simulink model "Final_Project_EEM_EKF_SIM"  (R2020a)
settings: Solver=ode45  StartTime=0  StopTime=t_runtime  FixedStep=clockt/4  RelTol=1e-3  AbsTol=1e-6
PreLoadFcn:
  | run(fullfile('Final_Project_EEM_SIM_init_params.m'));
StopFcn:
  | run('EKF_Simulation_Run_Plots_EEM.m');
values from neighbouring files (symbols this model uses):
  alph1 = Force*L_arm/I1    (= 0.055)    [Final_Project_EEM_SIM_init_params.m]
  alphs1 = 0.1*alph1    (= 0.0055)    [Final_Project_EEM_SIM_init_params.m]
  alphsu = 0.1*alphu    [Final_Project_EEM_SIM_init_params.m]
  alphsv = 0.1*alphv    [Final_Project_EEM_SIM_init_params.m]
  alphu = [sqrt(2) sqrt(2)]/2*[alph2 alph3]'    [Final_Project_EEM_SIM_init_params.m]
  alphv = [-sqrt(2) sqrt(2)]/2*[alph2 alph3]'    [Final_Project_EEM_SIM_init_params.m]
  clockt = 1/200    (= 0.005)    [Final_Project_EEM_SIM_init_params.m]
  DB = 0.345*pi/180    (= 0.00602138591938)    [Final_Project_EEM_SIM_init_params.m]
  delt = .1    (= 0.1)    [Final_Project_EEM_SIM_init_params.m]
  euler_0 = [-30 -10 -60]    [Final_Project_EEM_SIM_init_params.m]
  f_moon = .0012    (= 0.0012)    [Final_Project_EEM_SIM_init_params.m]
  Force = 100    [Final_Project_EEM_SIM_init_params.m]
  Inertia_0 = diag([I2,I3,I1],0)    [Final_Project_EEM_SIM_init_params.m]
  L_arm = 5.5    [Final_Project_EEM_SIM_init_params.m]
  lla_0 = [0.6, 23, 50000]    [Final_Project_EEM_SIM_init_params.m]
  mass_0 = 33296    [Final_Project_EEM_SIM_init_params.m]
  omega_moon = 2.7e-6    (= 2.7e-06)    [Final_Project_EEM_SIM_init_params.m]
  pqr_0 = [0.5730    0.5730    6.8080]    [Final_Project_EEM_SIM_init_params.m]
  r_moon_eq = 5702428    [Final_Project_EEM_SIM_init_params.m]
  tmin = 0.014    [Final_Project_EEM_SIM_init_params.m]
  vel_0 = angle2dcm(euler_0(3)*pi/180, euler_0(2)*pi/180, euler_0(1)*pi/180, 'ZYX')*vel    [Final_Project_EEM_SIM_init_params.m]
undefined symbols (not defined in the file or in its folder): deg, e0_0, e1_0, e2_0, e3_0, Newton, rad, Raphson, s
libraries: sharedtransform x5, sharedutil x5, aerolibtransform2 x4, shared6dofsys x3, aerolibconvert2 x3, vrlib x2, aerolibutil x1, aerolibgravity2 x1, aero_libdap x1
(part 2 of 3)

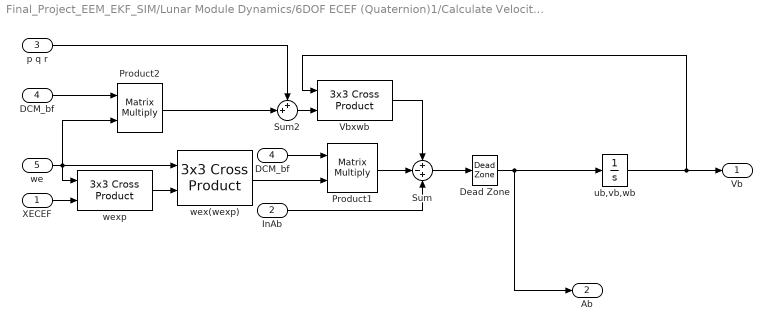
== system Final_Project_EEM_EKF_SIM/Lunar Module Dynamics/6DOF ECEF (Quaternion)1/Calculate Velocity in Body Axes ==
  XECEF : Inport
  InAb : Inport  Port=2
  p q r : Inport  Port=3
  DCM_bf : Inport  Port=4
  we : Inport  Port=5
  "DCM_bf " : InportShadow  Port=4
  Dead Zone : DeadZone  LowerValue=-eps  UpperValue=eps  SaturateOnIntegerOverflow=on
  Product1 : Product  Multiplication=Matrix(*)  RndMeth=Zero
  Product2 : Product  Multiplication=Matrix(*)  RndMeth=Zero
  Sum : Sum  Inputs=+-+  SaturateOnIntegerOverflow=on
  Sum2 : Sum  Inputs=++|  SaturateOnIntegerOverflow=on
  Vbxwb : sharedutil/3x3 Cross Product  aMode=aMode
      settings: SourceProductBaseCode=AE,PW,MT,VE,VP
  ub,vb,wb : Integrator  InitialCondition=Vm_0  ContinuousStateAttributes=Vm_statename
  wex(wexp) : sharedutil/3x3 Cross Product  aMode=aMode
      settings: SourceProductBaseCode=AE,PW,MT,VE,VP
  wexp : sharedutil/3x3 Cross Product  aMode=aMode
      settings: SourceProductBaseCode=AE,PW,MT,VE,VP
  Vb : Outport  VectorParamsAs1DForOutWhenUnconnected=off
  Ab : Outport  Port=2  PortDimensions=3  VectorParamsAs1DForOutWhenUnconnected=off
  wires:
  DCM_bf/1 -> Product1/1
  we/1 -> wex(wexp)/1, wexp/1, Product2/2
  InAb/1 -> Sum/3
  Vbxwb/1 -> Sum/1
  XECEF/1 -> wexp/2
  wex(wexp)/1 -> Product1/2
  wexp/1 -> wex(wexp)/2
  Product2/1 -> Sum2/2
  Sum2/1 -> Vbxwb/2
  Product1/1 -> Sum/2
  Sum/1 -> Dead Zone/1
  ub,vb,wb/1 -> Vbxwb/1, Vb/1
  "DCM_bf "/1 -> Product2/1
  p q r/1 -> Sum2/1
  Dead Zone/1 -> ub,vb,wb/1, Ab/1

== system Final_Project_EEM_EKF_SIM/Lunar Module Dynamics/6DOF ECEF (Quaternion)1/Celestial Longitude of Greenwich ==
  Initial Angle : Inport  Unit=rad
  Constant1 : Constant  Value=w_E
  Integrator : Integrator  ContinuousStateAttributes=LG_statename
  Sum : Sum  Inputs=|++
  Lambda : Outport  VectorParamsAs1DForOutWhenUnconnected=off
  wires:
  Initial Angle/1 -> Sum/1
  Integrator/1 -> Sum/2
  Constant1/1 -> Integrator/1  "we"
  Sum/1 -> Lambda/1

== system Final_Project_EEM_EKF_SIM/Lunar Module Dynamics/6DOF ECEF (Quaternion)1/ECEF to Inertial ==
  LG : Inport
  Create 3x3 Matrix : sharedutil/Create 3x3 Matrix  aMode=aMode
      settings: SourceProductBaseCode=AE,PW,MT,VE,VP
  Unary Minus : UnaryMinus
  Zero : Constant  Value=0
  Zero1 : Constant
  sincos : Trigonometry  Operator=sincos
  DCM_IF : Outport  VectorParamsAs1DForOutWhenUnconnected=off
  wires:
  LG/1 -> sincos/1
  Create 3x3 Matrix/1 -> DCM_IF/1
  Zero1/1 -> Create 3x3 Matrix/9
  Zero/1 -> Create 3x3 Matrix/8, Create 3x3 Matrix/7, Create 3x3 Matrix/6, Create 3x3 Matrix/3
  sincos/2 -> Create 3x3 Matrix/1, Create 3x3 Matrix/5
  sincos/1 -> Create 3x3 Matrix/4, Unary Minus/1
  Unary Minus/1 -> Create 3x3 Matrix/2

== system Final_Project_EEM_EKF_SIM/Lunar Module Dynamics/6DOF ECEF (Quaternion)1/Velocity Conversion ==
  in : Inport  Unit=ft/s
  Unit Conversion : UnitConversion
  out : Outport  VectorParamsAs1DForOutWhenUnconnected=off
  wires:
  in/1 -> Unit Conversion/1
  Unit Conversion/1 -> out/1

== system Final_Project_EEM_EKF_SIM/Lunar Module Dynamics/6DOF ECEF (Quaternion)1/Velocity Conversion1 ==
  in : Inport  Unit=ft/sec^2
  Unit Conversion : UnitConversion
  out : Outport  VectorParamsAs1DForOutWhenUnconnected=off
  wires:
  in/1 -> Unit Conversion/1
  Unit Conversion/1 -> out/1

== system Final_Project_EEM_EKF_SIM/Lunar Module Dynamics/6DOF ECEF (Quaternion)1/Velocity Conversion2 ==
  in : Inport  Unit=ft/s
  Unit Conversion : UnitConversion
  out : Outport  Unit=ft/s  VectorParamsAs1DForOutWhenUnconnected=off
  wires:
  in/1 -> Unit Conversion/1
  Unit Conversion/1 -> out/1

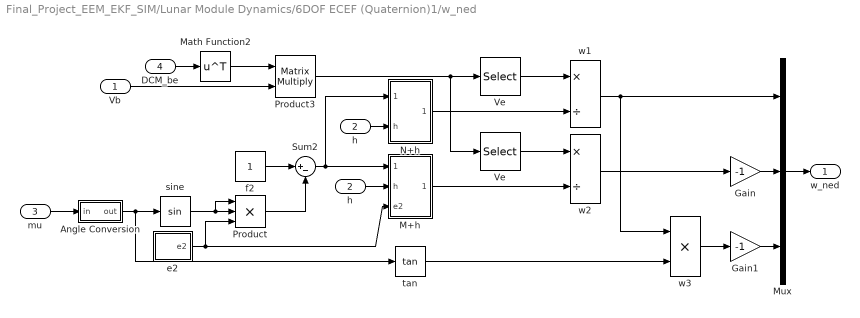
== system Final_Project_EEM_EKF_SIM/Lunar Module Dynamics/6DOF ECEF (Quaternion)1/w_ned ==
  Vb : Inport
  h : Inport  Port=2
  mu : Inport  Port=3
  DCM_be : Inport  Port=4
  Angle Conversion : Subsystem
  Gain : Gain  Gain=-1
  Gain1 : Gain  Gain=-1
  M+h : Subsystem
  Math Function2 : Math  Operator=transpose  SignedPower=on  SaturateOnIntegerOverflow=on
  Mux : Mux  Inputs=3
  N+h : Subsystem
  Product : Product  Inputs=3  RndMeth=Zero
  Product3 : Product  Multiplication=Matrix(*)  RndMeth=Zero
  Sum2 : Sum  Inputs=|+-
  Ve : Selector  InputPortWidth=3  IndexOptions=Index vector (dialog)  Indices=2  OutputSizes=1
  "Ve " : Selector  InputPortWidth=3  IndexOptions=Index vector (dialog)  Indices=1  OutputSizes=1
  e2 : Subsystem
  f2 : Constant
  "h " : InportShadow  Port=2
  sine : Trigonometry
  tan : Trigonometry  Operator=tan
  w1 : Product  Inputs=*/
  w2 : Product  Inputs=*/
  w3 : Product  Inputs=**
  w_ned : Outport  VectorParamsAs1DForOutWhenUnconnected=off
  wires:
  Angle Conversion/1(out) -> sine/1, tan/1
  Math Function2/1 -> Product3/1
  Vb/1 -> Product3/2
  DCM_be/1 -> Math Function2/1
  "h "/1 -> N+h/2(h)
  h/1 -> M+h/2(h)
  Product3/1 -> Ve/1, "Ve "/1
  mu/1 -> Angle Conversion/1(in)
  e2/1(e2) -> Product/3, M+h/3(e2)
  sine/1 -> Product/2, Product/1
  Product/1 -> Sum2/2
  f2/1 -> Sum2/1
  Sum2/1 -> N+h/1(den), M+h/1(den)
  Ve/1 -> w1/1
  N+h/1(N+h) -> w1/2
  "Ve "/1 -> w2/1
  M+h/1(M+h) -> w2/2
  w2/1 -> Gain/1
  tan/1 -> w3/2
  w1/1 -> w3/1, Mux/1
  w3/1 -> Gain1/1
  Gain/1 -> Mux/2
  Gain1/1 -> Mux/3
  Mux/1 -> w_ned/1

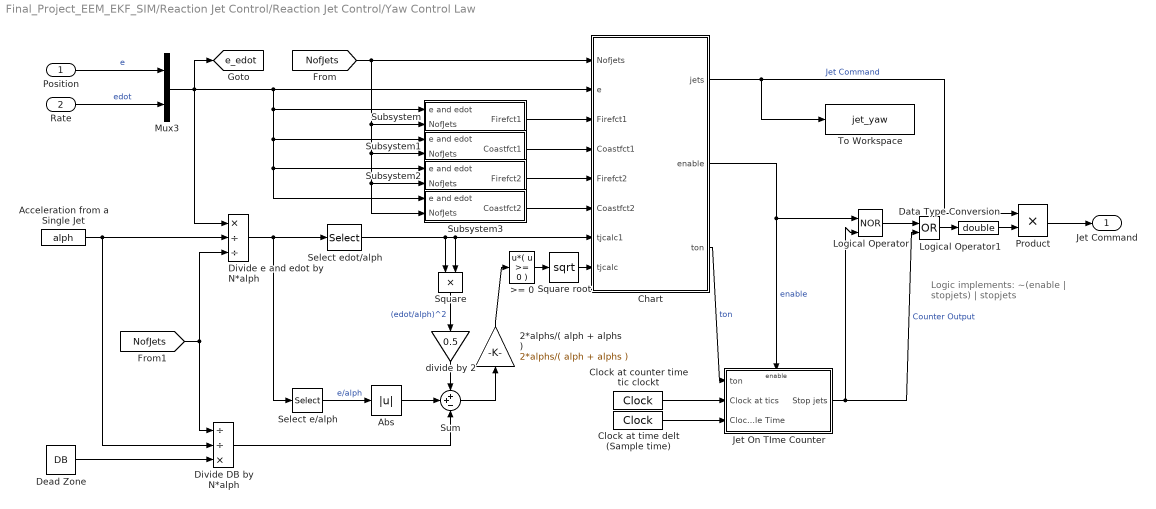
== system Final_Project_EEM_EKF_SIM/Reaction Jet Control/Reaction Jet Control/Yaw Control Law ==
  note: Logic implements:
      | ~(enable | stopjets) | stopjets
  Position : Inport  Unit=rad
  Rate : Inport  Port=2  Unit=rad/sec
  2*alphs/( alph + alphs ) : Gain  Gain=2*alphs/( alph + alphs )  SaturateOnIntegerOverflow=on  OutDataTypeStr=Inherit: Same as input  ParamDataTypeStr=Inherit: Same as input
  >= 0 : Fcn  Expr=u*( u >= 0 )
  Abs : Abs  SaturateOnIntegerOverflow=on
  Acceleration from a Single Jet : Constant  Value=alph
  Chart : Stateflow chart  TreatAsAtomicUnit=on
  Clock at counter time tic clockt : DigitalClock  SampleTime=clockt
  Clock at time delt (Sample time) : DigitalClock  SampleTime=delt
  Data Type Conversion : DataTypeConversion  OutDataTypeStr=double
  Dead Zone : Constant  Value=DB
  Divide e and edot by N*alph : Product  Inputs=*//  InputSameDT=on  RndMeth=Zero  SaturateOnIntegerOverflow=on  OutDataTypeStr=Inherit: Same as first input
  Divide DB by N*alph : Product  Inputs=//*  InputSameDT=on  RndMeth=Zero  SaturateOnIntegerOverflow=on  OutDataTypeStr=Inherit: Same as first input
  Jet On TIme Counter : Subsystem  TreatAsAtomicUnit=on
  Logical Operator : Logic  Operator=NOR  IconShape=distinctive  OutDataTypeStr=boolean
  Logical Operator1 : Logic  Operator=OR  IconShape=distinctive  OutDataTypeStr=boolean
  Mux3 : Mux  Inputs=2
  Product : Product  InputSameDT=on  RndMeth=Zero  SaturateOnIntegerOverflow=on  OutDataTypeStr=Inherit: Same as first input
  Select e/alph : Selector  InputPortWidth=2  IndexOptions=Index vector (dialog)  Indices=[1]  OutputSizes=1
  Select edot/alph : Selector  InputPortWidth=2  IndexOptions=Index vector (dialog)  Indices=[2]  OutputSizes=1
  Square : Product  InputSameDT=on  RndMeth=Zero  SaturateOnIntegerOverflow=on  OutDataTypeStr=Inherit: Same as first input
  Square root : Math  Operator=sqrt  SignedPower=on  SaturateOnIntegerOverflow=on
  Subsystem : Subsystem
  Subsystem1 : Subsystem
  Subsystem2 : Subsystem
  Subsystem3 : Subsystem
  Sum : Sum  Inputs=++-  InputSameDT=on  SaturateOnIntegerOverflow=on  OutDataTypeStr=Inherit: Same as first input
  To Workspace : ToWorkspace  VariableName=jet_yaw  SaveFormat=Timeseries  SampleTime=-1
  divide by 2 : Gain  Gain=0.5  SaturateOnIntegerOverflow=on  OutDataTypeStr=Inherit: Same as input  ParamDataTypeStr=Inherit: Same as input
  Jet Command : Outport  Unit=lbf  InitialOutput=0  VectorParamsAs1DForOutWhenUnconnected=off
  tag scope: e_edot=global
  wires:
  Data Type Conversion/1 -> Product/2
  >= 0/1 -> Square root/1
  2*alphs/( alph + alphs )/1 -> >= 0/1
  [NofJets] -> Subsystem3/2(NofJets), Subsystem2/2(NofJets), Subsystem1/2(NofJets), Subsystem/2(NofJets), Chart/1(Nofjets)
  Rate/1 -> Mux3/2  "edot"
  Position/1 -> Mux3/1  "e"
  Mux3/1 -> Divide e and edot by N*alph/1, Subsystem/1(e and edot), Subsystem1/1(e and edot), Subsystem2/1(e and edot), Subsystem3/1(e and edot), Chart/2(e), [e_edot]
  Square/1 -> divide by 2/1  "(edot/alph)^2"
  Square root/1 -> Chart/8(tjcalc)
  Chart/1(jets) -> To Workspace/1, Product/1  "Jet Command"
  Select edot/alph/1 -> Square/1, Chart/7(tjcalc1), Square/2
  Select e/alph/1 -> Abs/1  "e/alph"
  divide by 2/1 -> Sum/1
  Sum/1 -> 2*alphs/( alph + alphs )/1
  Abs/1 -> Sum/2
  Divide e and edot by N*alph/1 -> Select edot/alph/1, Select e/alph/1
  [NofJets] -> Divide e and edot by N*alph/3, Divide DB by N*alph/1
  Acceleration from a Single Jet/1 -> Divide DB by N*alph/2, Divide e and edot by N*alph/2
  Dead Zone/1 -> Divide DB by N*alph/3
  Divide DB by N*alph/1 -> Sum/3
  Chart/2(enable) -> Jet On TIme Counter/Enable, Logical Operator/1  "enable"
  Logical Operator1/1 -> Data Type Conversion/1
  Chart/3(ton) -> Jet On TIme Counter/1(ton)  "ton"
  Clock at counter time tic clockt/1 -> Jet On TIme Counter/2(Clock at tics)
  Clock at time delt (Sample time)/1 -> Jet On TIme Counter/3(Clock at Sample Time)
  Jet On TIme Counter/1(Stop jets) -> Logical Operator/2, Logical Operator1/2  "Counter Output"
  Logical Operator/1 -> Logical Operator1/1
  Subsystem3/1(Coastfct2) -> Chart/6(Coastfct2)
  Subsystem2/1(Firefct2) -> Chart/5(Firefct2)
  Subsystem1/1(Coastfct1) -> Chart/4(Coastfct1)
  Subsystem/1(Firefct1) -> Chart/3(Firefct1)
  Product/1 -> Jet Command/1

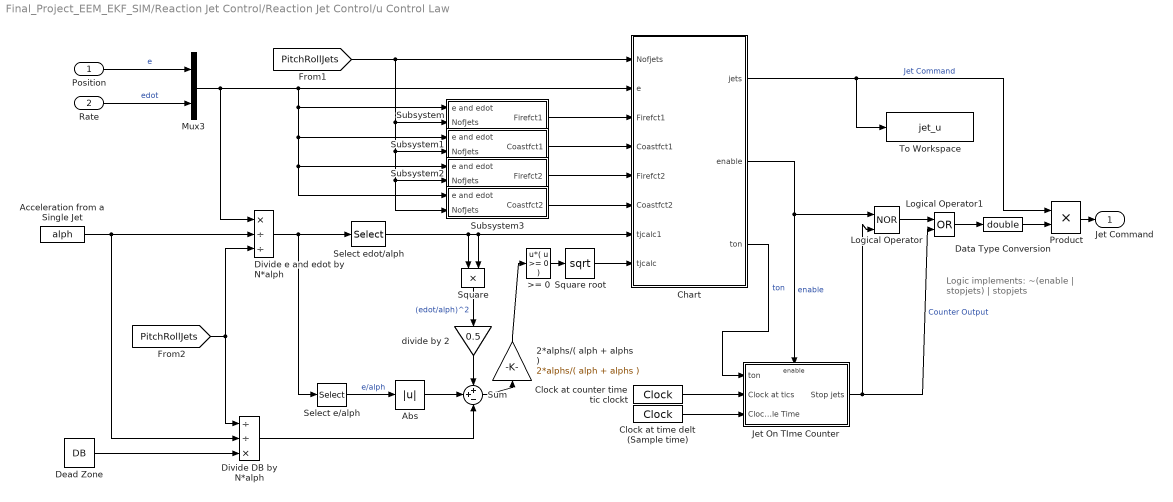
== system Final_Project_EEM_EKF_SIM/Reaction Jet Control/Reaction Jet Control/u Control Law ==
  note: Logic implements:
      | ~(enable | stopjets) | stopjets
  Position : Inport  Unit=rad
  Rate : Inport  Port=2  Unit=rad/sec
  2*alphs/( alph + alphs ) : Gain  Gain=2*alphs/( alph + alphs )  SaturateOnIntegerOverflow=on  OutDataTypeStr=Inherit: Same as input  ParamDataTypeStr=Inherit: Same as input
  >= 0 : Fcn  Expr=u*( u >= 0 )
  Abs : Abs  SaturateOnIntegerOverflow=on
  Acceleration from a Single Jet : Constant  Value=alph
  Chart : Stateflow chart  TreatAsAtomicUnit=on
  Clock at counter time tic clockt : DigitalClock  SampleTime=clockt
  Clock at time delt (Sample time) : DigitalClock  SampleTime=delt
  Data Type Conversion : DataTypeConversion  OutDataTypeStr=double
  Dead Zone : Constant  Value=DB
  Divide e and edot by N*alph : Product  Inputs=*//  InputSameDT=on  RndMeth=Zero  SaturateOnIntegerOverflow=on  OutDataTypeStr=Inherit: Same as first input
  Divide DB by N*alph : Product  Inputs=//*  InputSameDT=on  RndMeth=Zero  SaturateOnIntegerOverflow=on  OutDataTypeStr=Inherit: Same as first input
  Jet On TIme Counter : Subsystem  TreatAsAtomicUnit=on
  Logical Operator : Logic  Operator=NOR  IconShape=distinctive  OutDataTypeStr=boolean
  Logical Operator1 : Logic  Operator=OR  IconShape=distinctive  OutDataTypeStr=boolean
  Mux3 : Mux  Inputs=2
  Product : Product  InputSameDT=on  RndMeth=Zero  SaturateOnIntegerOverflow=on  OutDataTypeStr=Inherit: Same as first input
  Select e/alph : Selector  InputPortWidth=2  IndexOptions=Index vector (dialog)  Indices=[1]  OutputSizes=1
  Select edot/alph : Selector  InputPortWidth=2  IndexOptions=Index vector (dialog)  Indices=[2]  OutputSizes=1
  Square : Product  InputSameDT=on  RndMeth=Zero  SaturateOnIntegerOverflow=on  OutDataTypeStr=Inherit: Same as first input
  Square root : Math  Operator=sqrt  SignedPower=on  SaturateOnIntegerOverflow=on
  Subsystem : Subsystem
  Subsystem1 : Subsystem
  Subsystem2 : Subsystem
  Subsystem3 : Subsystem
  Sum : Sum  Inputs=++-  InputSameDT=on  SaturateOnIntegerOverflow=on  OutDataTypeStr=Inherit: Same as first input
  To Workspace : ToWorkspace  VariableName=jet_u  SaveFormat=Timeseries  SampleTime=-1
  divide by 2 : Gain  Gain=0.5  SaturateOnIntegerOverflow=on  OutDataTypeStr=Inherit: Same as input  ParamDataTypeStr=Inherit: Same as input
  Jet Command : Outport  Unit=lbf  InitialOutput=0  VectorParamsAs1DForOutWhenUnconnected=off
  wires:
  Data Type Conversion/1 -> Product/2
  >= 0/1 -> Square root/1
  2*alphs/( alph + alphs )/1 -> >= 0/1
  Product/1 -> Jet Command/1
  Subsystem/1(Firefct1) -> Chart/3(Firefct1)
  Subsystem1/1(Coastfct1) -> Chart/4(Coastfct1)
  Subsystem2/1(Firefct2) -> Chart/5(Firefct2)
  Subsystem3/1(Coastfct2) -> Chart/6(Coastfct2)
  Logical Operator/1 -> Logical Operator1/1
  Jet On TIme Counter/1(Stop jets) -> Logical Operator1/2, Logical Operator/2  "Counter Output"
  Clock at time delt (Sample time)/1 -> Jet On TIme Counter/3(Clock at Sample Time)
  Clock at counter time tic clockt/1 -> Jet On TIme Counter/2(Clock at tics)
  Chart/3(ton) -> Jet On TIme Counter/1(ton)  "ton"
  Logical Operator1/1 -> Data Type Conversion/1
  Chart/2(enable) -> Jet On TIme Counter/Enable, Logical Operator/1  "enable"
  Divide DB by N*alph/1 -> Sum/3
  Dead Zone/1 -> Divide DB by N*alph/3
  Acceleration from a Single Jet/1 -> Divide DB by N*alph/2, Divide e and edot by N*alph/2
  [PitchRollJets] -> Divide DB by N*alph/1, Divide e and edot by N*alph/3
  Divide e and edot by N*alph/1 -> Select e/alph/1, Select edot/alph/1
  Abs/1 -> Sum/2
  Sum/1 -> 2*alphs/( alph + alphs )/1
  divide by 2/1 -> Sum/1
  Select e/alph/1 -> Abs/1  "e/alph"
  Select edot/alph/1 -> Square/2, Chart/7(tjcalc1), Square/1
  Square root/1 -> Chart/8(tjcalc)
  Square/1 -> divide by 2/1  "(edot/alph)^2"
  Mux3/1 -> Divide e and edot by N*alph/1, Subsystem3/1(e and edot), Subsystem2/1(e and edot), Subsystem1/1(e and edot), Subsystem/1(e and edot), Chart/2(e)
  Position/1 -> Mux3/1  "e"
  Rate/1 -> Mux3/2  "edot"
  [PitchRollJets] -> Chart/1(Nofjets), Subsystem/2(NofJets), Subsystem1/2(NofJets), Subsystem2/2(NofJets), Subsystem3/2(NofJets)
  Chart/1(jets) -> To Workspace/1, Product/1  "Jet Command"

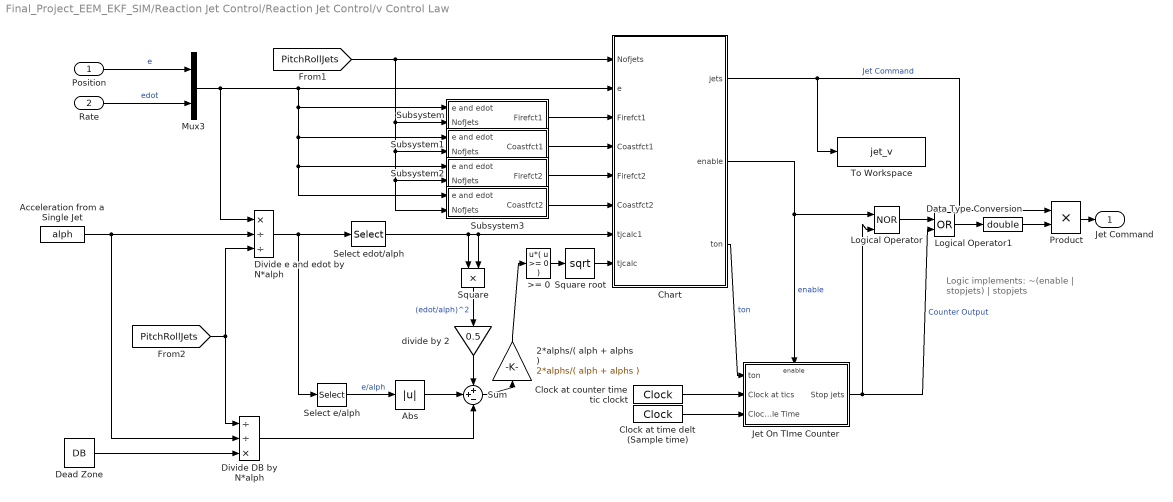
== system Final_Project_EEM_EKF_SIM/Reaction Jet Control/Reaction Jet Control/v Control Law ==
  note: Logic implements:
      | ~(enable | stopjets) | stopjets
  Position : Inport  Unit=rad
  Rate : Inport  Port=2  Unit=rad/sec
  2*alphs/( alph + alphs ) : Gain  Gain=2*alphs/( alph + alphs )  SaturateOnIntegerOverflow=on  OutDataTypeStr=Inherit: Same as input  ParamDataTypeStr=Inherit: Same as input
  >= 0 : Fcn  Expr=u*( u >= 0 )
  Abs : Abs  SaturateOnIntegerOverflow=on
  Acceleration from a Single Jet : Constant  Value=alph
  Chart : Stateflow chart  TreatAsAtomicUnit=on
  Clock at counter time tic clockt : DigitalClock  SampleTime=clockt
  Clock at time delt (Sample time) : DigitalClock  SampleTime=delt
  Data Type Conversion : DataTypeConversion  OutDataTypeStr=double
  Dead Zone : Constant  Value=DB
  Divide e and edot by N*alph : Product  Inputs=*//  InputSameDT=on  RndMeth=Zero  SaturateOnIntegerOverflow=on  OutDataTypeStr=Inherit: Same as first input
  Divide DB by N*alph : Product  Inputs=//*  InputSameDT=on  RndMeth=Zero  SaturateOnIntegerOverflow=on  OutDataTypeStr=Inherit: Same as first input
  Jet On TIme Counter : Subsystem  TreatAsAtomicUnit=on
  Logical Operator : Logic  Operator=NOR  IconShape=distinctive  OutDataTypeStr=boolean
  Logical Operator1 : Logic  Operator=OR  IconShape=distinctive  OutDataTypeStr=boolean
  Mux3 : Mux  Inputs=2
  Product : Product  InputSameDT=on  RndMeth=Zero  SaturateOnIntegerOverflow=on  OutDataTypeStr=Inherit: Same as first input
  Select e/alph : Selector  InputPortWidth=2  IndexOptions=Index vector (dialog)  Indices=[1]  OutputSizes=1
  Select edot/alph : Selector  InputPortWidth=2  IndexOptions=Index vector (dialog)  Indices=[2]  OutputSizes=1
  Square : Product  InputSameDT=on  RndMeth=Zero  SaturateOnIntegerOverflow=on  OutDataTypeStr=Inherit: Same as first input
  Square root : Math  Operator=sqrt  SignedPower=on  SaturateOnIntegerOverflow=on
  Subsystem : Subsystem
  Subsystem1 : Subsystem
  Subsystem2 : Subsystem
  Subsystem3 : Subsystem
  Sum : Sum  Inputs=++-  InputSameDT=on  SaturateOnIntegerOverflow=on  OutDataTypeStr=Inherit: Same as first input
  To Workspace : ToWorkspace  VariableName=jet_v  SaveFormat=Timeseries  SampleTime=-1
  divide by 2 : Gain  Gain=0.5  SaturateOnIntegerOverflow=on  OutDataTypeStr=Inherit: Same as input  ParamDataTypeStr=Inherit: Same as input
  Jet Command : Outport  Unit=lbf  InitialOutput=0  VectorParamsAs1DForOutWhenUnconnected=off
  wires:
  Data Type Conversion/1 -> Product/2
  >= 0/1 -> Square root/1
  2*alphs/( alph + alphs )/1 -> >= 0/1
  Product/1 -> Jet Command/1
  Subsystem/1(Firefct1) -> Chart/3(Firefct1)
  Subsystem1/1(Coastfct1) -> Chart/4(Coastfct1)
  Subsystem2/1(Firefct2) -> Chart/5(Firefct2)
  Subsystem3/1(Coastfct2) -> Chart/6(Coastfct2)
  Logical Operator/1 -> Logical Operator1/1
  Jet On TIme Counter/1(Stop jets) -> Logical Operator1/2, Logical Operator/2  "Counter Output"
  Clock at time delt (Sample time)/1 -> Jet On TIme Counter/3(Clock at Sample Time)
  Clock at counter time tic clockt/1 -> Jet On TIme Counter/2(Clock at tics)
  Chart/3(ton) -> Jet On TIme Counter/1(ton)  "ton"
  Logical Operator1/1 -> Data Type Conversion/1
  Chart/2(enable) -> Logical Operator/1, Jet On TIme Counter/Enable  "enable"
  Divide DB by N*alph/1 -> Sum/3
  Dead Zone/1 -> Divide DB by N*alph/3
  Acceleration from a Single Jet/1 -> Divide DB by N*alph/2, Divide e and edot by N*alph/2
  [PitchRollJets] -> Divide DB by N*alph/1, Divide e and edot by N*alph/3
  Divide e and edot by N*alph/1 -> Select e/alph/1, Select edot/alph/1
  Abs/1 -> Sum/2
  Sum/1 -> 2*alphs/( alph + alphs )/1
  divide by 2/1 -> Sum/1
  Select e/alph/1 -> Abs/1  "e/alph"
  Select edot/alph/1 -> Square/2, Chart/7(tjcalc1), Square/1
  Chart/1(jets) -> To Workspace/1, Product/1  "Jet Command"
  Square root/1 -> Chart/8(tjcalc)
  Square/1 -> divide by 2/1  "(edot/alph)^2"
  Mux3/1 -> Divide e and edot by N*alph/1, Subsystem3/1(e and edot), Subsystem2/1(e and edot), Subsystem1/1(e and edot), Subsystem/1(e and edot), Chart/2(e)
  Position/1 -> Mux3/1  "e"
  Rate/1 -> Mux3/2  "edot"
  [PitchRollJets] -> Chart/1(Nofjets), Subsystem/2(NofJets), Subsystem1/2(NofJets), Subsystem2/2(NofJets), Subsystem3/2(NofJets)

== system Final_Project_EEM_EKF_SIM/Lunar Module Dynamics/6DOF ECEF (Quaternion)1/w_ned/Angle Conversion ==
  in : Inport  Unit=deg
  Unit Conversion : UnitConversion
  out : Outport  Unit=rad  VectorParamsAs1DForOutWhenUnconnected=off
  wires:
  in/1 -> Unit Conversion/1
  Unit Conversion/1 -> out/1

== system Final_Project_EEM_EKF_SIM/Lunar Module Dynamics/6DOF ECEF (Quaternion)1/w_ned/M+h ==
  den : Inport
  h : Inport  Port=2
  e2 : Inport  Port=3
  M : Product  Inputs=**/
  Math Function : Math  Operator=pow  SignedPower=on  SaturateOnIntegerOverflow=on
  Sum : Sum  Inputs=|+-
  Sum1 : Sum  Inputs=|++  SaturateOnIntegerOverflow=on
  f : Constant
  f1 : Constant  Value=R
  f3 : Constant  Value=1.5
  M+h : Outport  VectorParamsAs1DForOutWhenUnconnected=off
  wires:
  Sum1/1 -> M+h/1
  den/1 -> Math Function/1
  e2/1 -> Sum/2
  f/1 -> Sum/1
  Sum/1 -> M/2
  f1/1 -> M/1
  Math Function/1 -> M/3
  f3/1 -> Math Function/2
  M/1 -> Sum1/1
  h/1 -> Sum1/2

== system Final_Project_EEM_EKF_SIM/Lunar Module Dynamics/6DOF ECEF (Quaternion)1/w_ned/N+h ==
  den : Inport
  h : Inport  Port=2
  N : Product  Inputs=*/
  Sum4 : Sum  Inputs=|++  SaturateOnIntegerOverflow=on
  f4 : Constant  Value=R
  sqrt : Sqrt  AlgorithmType=Newton-Raphson  SaturateOnIntegerOverflow=on
  N+h : Outport  VectorParamsAs1DForOutWhenUnconnected=off
  wires:
  Sum4/1 -> N+h/1
  den/1 -> sqrt/1
  sqrt/1 -> N/2
  f4/1 -> N/1
  h/1 -> Sum4/2
  N/1 -> Sum4/1

== system Final_Project_EEM_EKF_SIM/Lunar Module Dynamics/6DOF ECEF (Quaternion)1/w_ned/e2 ==
  Constant : Constant  Value=F
  Product3 : Product  RndMeth=Zero
  Sum : Sum  Inputs=-+
  Sum2 : Sum  Inputs=|-+
  f : Constant
  e2 : Outport  VectorParamsAs1DForOutWhenUnconnected=off
  wires:
  Constant/1 -> Sum/1
  f/1 -> Sum/2, Sum2/2
  Sum/1 -> Product3/2, Product3/1
  Product3/1 -> Sum2/1
  Sum2/1 -> e2/1

== system Final_Project_EEM_EKF_SIM/Reaction Jet Control/Reaction Jet Control/Yaw Control Law/Jet On TIme Counter ==
  ton : Inport
  Clock at tics : Inport  Port=2
  Clock at Sample Time : Inport  Port=3
  Enable : EnablePort  StatesWhenEnabling=reset
  Constant : Constant  Value=0
  Relational Operator : RelationalOperator  Operator=>  OutDataTypeStr=boolean  RndMeth=Nearest  InputSameDT=on
  Sum : Sum  Inputs=|+-  InputSameDT=on  SaturateOnIntegerOverflow=on  OutDataTypeStr=Inherit: Same as first input
  Sum1 : Sum  Inputs=|+-  InputSameDT=on  SaturateOnIntegerOverflow=on  OutDataTypeStr=Inherit: Same as first input
  Stop jets : Outport  VectorParamsAs1DForOutWhenUnconnected=off
  wires:
  Constant/1 -> Relational Operator/2
  ton/1 -> Sum/1  "ton"
  Clock at tics/1 -> Sum1/1  "Time in clockt multiples"
  Clock at Sample Time/1 -> Sum1/2  "Time in delt multiples"
  Sum1/1 -> Sum/2  "Time after last sample in clock tics"
  Sum/1 -> Relational Operator/1  "Count down of ton"
  Relational Operator/1 -> Stop jets/1  "Stop Command"

== system Final_Project_EEM_EKF_SIM/Reaction Jet Control/Reaction Jet Control/Yaw Control Law/Subsystem ==
  note: Firefct1
      | This function establishes when the jets are to be fired in a negative sense
      | Firefct1 = e + edot ^2/(2*N*alph) - DB
  e and edot : Inport
  NofJets : Inport  Port=2
  1/(2*alph) : Gain  Gain=1/(2*alph)  SaturateOnIntegerOverflow=on  OutDataTypeStr=Inherit: Same as input  ParamDataTypeStr=Inherit: Same as input
  Constant2 : Constant  Value=DB
  Select e : Selector  InputPortWidth=2  IndexOptions=Index vector (dialog)  Indices=[1]  OutputSizes=1
  Select edot : Selector  InputPortWidth=2  IndexOptions=Index vector (dialog)  Indices=[2]  OutputSizes=1
  Sum1 : Sum  Inputs=-++  InputSameDT=on  SaturateOnIntegerOverflow=on  OutDataTypeStr=Inherit: Same as first input
  edot^2 : Product  Inputs=/**  InputSameDT=on  RndMeth=Zero  SaturateOnIntegerOverflow=on  OutDataTypeStr=Inherit: Same as first input
  Firefct1 : Outport  VectorParamsAs1DForOutWhenUnconnected=off
  wires:
  edot^2/1 -> 1/(2*alph)/1  "edot^2"
  Select edot/1 -> edot^2/2, edot^2/3  "edot"
  NofJets/1 -> edot^2/1
  e and edot/1 -> Select e/1, Select edot/1
  1/(2*alph)/1 -> Sum1/3
  Constant2/1 -> Sum1/1
  Select e/1 -> Sum1/2  "e"
  Sum1/1 -> Firefct1/1

== system Final_Project_EEM_EKF_SIM/Reaction Jet Control/Reaction Jet Control/Yaw Control Law/Subsystem1 ==
  note: Coastfct1
      | This function establishes when the jets are to be turned off (coasting)
      | Coastfct1 = e - edot ^2/(2*N*alphs) - DB
  e and edot : Inport
  NofJets : Inport  Port=2
  1/(2*alph) : Gain  Gain=1/(2*alphs)  SaturateOnIntegerOverflow=on  OutDataTypeStr=Inherit: Same as input  ParamDataTypeStr=Inherit: Same as input
  Constant2 : Constant  Value=DB
  Select e : Selector  InputPortWidth=2  IndexOptions=Index vector (dialog)  Indices=[1]  OutputSizes=1
  Select edot : Selector  InputPortWidth=2  IndexOptions=Index vector (dialog)  Indices=[2]  OutputSizes=1
  Sum1 : Sum  Inputs=-+-  InputSameDT=on  SaturateOnIntegerOverflow=on  OutDataTypeStr=Inherit: Same as first input
  edot^2 : Product  Inputs=/**  InputSameDT=on  RndMeth=Zero  SaturateOnIntegerOverflow=on  OutDataTypeStr=Inherit: Same as first input
  Coastfct1 : Outport  VectorParamsAs1DForOutWhenUnconnected=off
  wires:
  Sum1/1 -> Coastfct1/1
  Select e/1 -> Sum1/2  "e"
  Constant2/1 -> Sum1/1
  1/(2*alph)/1 -> Sum1/3
  e and edot/1 -> Select edot/1, Select e/1
  NofJets/1 -> edot^2/1
  Select edot/1 -> edot^2/3, edot^2/2  "edot"
  edot^2/1 -> 1/(2*alph)/1  "edot^2"

== system Final_Project_EEM_EKF_SIM/Reaction Jet Control/Reaction Jet Control/Yaw Control Law/Subsystem2 ==
  note: Firefct2
      | This function establishes when the jets are to be fired in a positive sense
      | Firefct2 = e - edot ^2/(2*N*alph) + DB
  e and edot : Inport
  NofJets : Inport  Port=2
  1/(2*alph) : Gain  Gain=1/(2*alph)  SaturateOnIntegerOverflow=on  OutDataTypeStr=Inherit: Same as input  ParamDataTypeStr=Inherit: Same as input
  Constant2 : Constant  Value=DB
  Select e : Selector  InputPortWidth=2  IndexOptions=Index vector (dialog)  Indices=[1]  OutputSizes=1
  Select edot : Selector  InputPortWidth=2  IndexOptions=Index vector (dialog)  Indices=[2]  OutputSizes=1
  Sum1 : Sum  Inputs=++-  InputSameDT=on  SaturateOnIntegerOverflow=on  OutDataTypeStr=Inherit: Same as first input
  edot^2 : Product  Inputs=/**  InputSameDT=on  RndMeth=Zero  SaturateOnIntegerOverflow=on  OutDataTypeStr=Inherit: Same as first input
  Firefct2 : Outport  VectorParamsAs1DForOutWhenUnconnected=off
  wires:
  edot^2/1 -> 1/(2*alph)/1  "edot^2"
  Select edot/1 -> edot^2/2, edot^2/3  "edot"
  NofJets/1 -> edot^2/1
  e and edot/1 -> Select e/1, Select edot/1
  1/(2*alph)/1 -> Sum1/3
  Constant2/1 -> Sum1/1
  Select e/1 -> Sum1/2  "e"
  Sum1/1 -> Firefct2/1

== system Final_Project_EEM_EKF_SIM/Reaction Jet Control/Reaction Jet Control/Yaw Control Law/Subsystem3 ==
  note: Coastfct2
      | This function establishes when the jets are to be turned off (coasting)
      | Coastfct1 = e + edot ^2/(2*N*alphs) + DB
  e and edot : Inport
  NofJets : Inport  Port=2
  1/(2*alph) : Gain  Gain=1/(2*alphs)  SaturateOnIntegerOverflow=on  OutDataTypeStr=Inherit: Same as input  ParamDataTypeStr=Inherit: Same as input
  Constant2 : Constant  Value=DB
  Select e : Selector  InputPortWidth=2  IndexOptions=Index vector (dialog)  Indices=[1]  OutputSizes=1
  Select edot : Selector  InputPortWidth=2  IndexOptions=Index vector (dialog)  Indices=[2]  OutputSizes=1
  Sum1 : Sum  Inputs=+++  InputSameDT=on  SaturateOnIntegerOverflow=on  OutDataTypeStr=Inherit: Same as first input
  edot^2 : Product  Inputs=/**  InputSameDT=on  RndMeth=Zero  SaturateOnIntegerOverflow=on  OutDataTypeStr=Inherit: Same as first input
  Coastfct2 : Outport  VectorParamsAs1DForOutWhenUnconnected=off
  wires:
  edot^2/1 -> 1/(2*alph)/1  "edot^2"
  Select edot/1 -> edot^2/2, edot^2/3  "edot"
  NofJets/1 -> edot^2/1
  e and edot/1 -> Select e/1, Select edot/1
  1/(2*alph)/1 -> Sum1/3
  Constant2/1 -> Sum1/1
  Select e/1 -> Sum1/2  "e"
  Sum1/1 -> Coastfct2/1

== system Final_Project_EEM_EKF_SIM/Reaction Jet Control/Reaction Jet Control/u Control Law/Jet On TIme Counter ==
  ton : Inport
  Clock at tics : Inport  Port=2
  Clock at Sample Time : Inport  Port=3
  Enable : EnablePort  StatesWhenEnabling=reset
  Constant : Constant  Value=0
  Relational Operator : RelationalOperator  Operator=>  OutDataTypeStr=boolean  RndMeth=Nearest  InputSameDT=on
  Sum : Sum  Inputs=|+-  InputSameDT=on  SaturateOnIntegerOverflow=on  OutDataTypeStr=Inherit: Same as first input
  Sum1 : Sum  Inputs=|+-  InputSameDT=on  SaturateOnIntegerOverflow=on  OutDataTypeStr=Inherit: Same as first input
  Stop jets : Outport  VectorParamsAs1DForOutWhenUnconnected=off
  wires:
  Relational Operator/1 -> Stop jets/1  "Stop Command"
  Sum/1 -> Relational Operator/1  "Count down of ton"
  Sum1/1 -> Sum/2  "Time after last sample in clock tics"
  Clock at Sample Time/1 -> Sum1/2  "Time in delt multiples"
  Clock at tics/1 -> Sum1/1  "Time in clockt multiples"
  ton/1 -> Sum/1  "ton"
  Constant/1 -> Relational Operator/2

== system Final_Project_EEM_EKF_SIM/Reaction Jet Control/Reaction Jet Control/u Control Law/Subsystem ==
  note: Firefct1
      | This function establishes when the jets are to be fired in a negative sense
      | Firefct1 = e + edot ^2/(2*N*alph) - DB
  e and edot : Inport
  NofJets : Inport  Port=2
  1/(2*alph) : Gain  Gain=1/(2*alph)  SaturateOnIntegerOverflow=on  OutDataTypeStr=Inherit: Same as input  ParamDataTypeStr=Inherit: Same as input
  Constant2 : Constant  Value=DB
  Select e : Selector  InputPortWidth=2  IndexOptions=Index vector (dialog)  Indices=[1]  OutputSizes=1
  Select edot : Selector  InputPortWidth=2  IndexOptions=Index vector (dialog)  Indices=[2]  OutputSizes=1
  Sum1 : Sum  Inputs=-++  InputSameDT=on  SaturateOnIntegerOverflow=on  OutDataTypeStr=Inherit: Same as first input
  edot^2 : Product  Inputs=/**  InputSameDT=on  RndMeth=Zero  SaturateOnIntegerOverflow=on  OutDataTypeStr=Inherit: Same as first input
  Firefct1 : Outport  VectorParamsAs1DForOutWhenUnconnected=off
  wires:
  Sum1/1 -> Firefct1/1
  Select e/1 -> Sum1/2  "e"
  Constant2/1 -> Sum1/1
  1/(2*alph)/1 -> Sum1/3
  e and edot/1 -> Select edot/1, Select e/1
  NofJets/1 -> edot^2/1
  Select edot/1 -> edot^2/3, edot^2/2  "edot"
  edot^2/1 -> 1/(2*alph)/1  "edot^2"

== system Final_Project_EEM_EKF_SIM/Reaction Jet Control/Reaction Jet Control/u Control Law/Subsystem1 ==
  note: Coastfct1
      | This function establishes when the jets are to be turned off (coasting)
      | Coastfct1 = e - edot ^2/(2*N*alphs) - DB
  e and edot : Inport
  NofJets : Inport  Port=2
  1/(2*alph) : Gain  Gain=1/(2*alphs)  SaturateOnIntegerOverflow=on  OutDataTypeStr=Inherit: Same as input  ParamDataTypeStr=Inherit: Same as input
  Constant2 : Constant  Value=DB
  Select e : Selector  InputPortWidth=2  IndexOptions=Index vector (dialog)  Indices=[1]  OutputSizes=1
  Select edot : Selector  InputPortWidth=2  IndexOptions=Index vector (dialog)  Indices=[2]  OutputSizes=1
  Sum1 : Sum  Inputs=-+-  InputSameDT=on  SaturateOnIntegerOverflow=on  OutDataTypeStr=Inherit: Same as first input
  edot^2 : Product  Inputs=/**  InputSameDT=on  RndMeth=Zero  SaturateOnIntegerOverflow=on  OutDataTypeStr=Inherit: Same as first input
  Coastfct1 : Outport  VectorParamsAs1DForOutWhenUnconnected=off
  wires:
  edot^2/1 -> 1/(2*alph)/1  "edot^2"
  Select edot/1 -> edot^2/2, edot^2/3  "edot"
  NofJets/1 -> edot^2/1
  e and edot/1 -> Select e/1, Select edot/1
  1/(2*alph)/1 -> Sum1/3
  Constant2/1 -> Sum1/1
  Select e/1 -> Sum1/2  "e"
  Sum1/1 -> Coastfct1/1

== system Final_Project_EEM_EKF_SIM/Reaction Jet Control/Reaction Jet Control/u Control Law/Subsystem2 ==
  note: Firefct2
      | This function establishes when the jets are to be fired in a positive sense
      | Firefct2 = e - edot ^2/(2*N*alph) + DB
  e and edot : Inport
  NofJets : Inport  Port=2
  1/(2*alph) : Gain  Gain=1/(2*alph)  SaturateOnIntegerOverflow=on  OutDataTypeStr=Inherit: Same as input  ParamDataTypeStr=Inherit: Same as input
  Constant2 : Constant  Value=DB
  Select e : Selector  InputPortWidth=2  IndexOptions=Index vector (dialog)  Indices=[1]  OutputSizes=1
  Select edot : Selector  InputPortWidth=2  IndexOptions=Index vector (dialog)  Indices=[2]  OutputSizes=1
  Sum1 : Sum  Inputs=++-  InputSameDT=on  SaturateOnIntegerOverflow=on  OutDataTypeStr=Inherit: Same as first input
  edot^2 : Product  Inputs=/**  InputSameDT=on  RndMeth=Zero  SaturateOnIntegerOverflow=on  OutDataTypeStr=Inherit: Same as first input
  Firefct2 : Outport  VectorParamsAs1DForOutWhenUnconnected=off
  wires:
  Sum1/1 -> Firefct2/1
  Select e/1 -> Sum1/2  "e"
  Constant2/1 -> Sum1/1
  1/(2*alph)/1 -> Sum1/3
  e and edot/1 -> Select edot/1, Select e/1
  NofJets/1 -> edot^2/1
  Select edot/1 -> edot^2/3, edot^2/2  "edot"
  edot^2/1 -> 1/(2*alph)/1  "edot^2"

== system Final_Project_EEM_EKF_SIM/Reaction Jet Control/Reaction Jet Control/u Control Law/Subsystem3 ==
  note: Coastfct2
      | This function establishes when the jets are to be turned off (coasting)
      | Coastfct1 = e + edot ^2/(2*N*alphs) + DB
  e and edot : Inport
  NofJets : Inport  Port=2
  1/(2*alph) : Gain  Gain=1/(2*alphs)  SaturateOnIntegerOverflow=on  OutDataTypeStr=Inherit: Same as input  ParamDataTypeStr=Inherit: Same as input
  Constant2 : Constant  Value=DB
  Select e : Selector  InputPortWidth=2  IndexOptions=Index vector (dialog)  Indices=[1]  OutputSizes=1
  Select edot : Selector  InputPortWidth=2  IndexOptions=Index vector (dialog)  Indices=[2]  OutputSizes=1
  Sum1 : Sum  Inputs=+++  InputSameDT=on  SaturateOnIntegerOverflow=on  OutDataTypeStr=Inherit: Same as first input
  edot^2 : Product  Inputs=/**  InputSameDT=on  RndMeth=Zero  SaturateOnIntegerOverflow=on  OutDataTypeStr=Inherit: Same as first input
  Coastfct2 : Outport  VectorParamsAs1DForOutWhenUnconnected=off
  wires:
  Sum1/1 -> Coastfct2/1
  Select e/1 -> Sum1/2  "e"
  Constant2/1 -> Sum1/1
  1/(2*alph)/1 -> Sum1/3
  e and edot/1 -> Select edot/1, Select e/1
  NofJets/1 -> edot^2/1
  Select edot/1 -> edot^2/3, edot^2/2  "edot"
  edot^2/1 -> 1/(2*alph)/1  "edot^2"

== system Final_Project_EEM_EKF_SIM/Reaction Jet Control/Reaction Jet Control/v Control Law/Jet On TIme Counter ==
  ton : Inport
  Clock at tics : Inport  Port=2
  Clock at Sample Time : Inport  Port=3
  Enable : EnablePort  StatesWhenEnabling=reset
  Constant : Constant  Value=0
  Relational Operator : RelationalOperator  Operator=>  OutDataTypeStr=boolean  RndMeth=Nearest  InputSameDT=on
  Sum : Sum  Inputs=|+-  InputSameDT=on  SaturateOnIntegerOverflow=on  OutDataTypeStr=Inherit: Same as first input
  Sum1 : Sum  Inputs=|+-  InputSameDT=on  SaturateOnIntegerOverflow=on  OutDataTypeStr=Inherit: Same as first input
  Stop jets : Outport  VectorParamsAs1DForOutWhenUnconnected=off
  wires:
  Relational Operator/1 -> Stop jets/1  "Stop Command"
  Sum/1 -> Relational Operator/1  "Count down of ton"
  Sum1/1 -> Sum/2  "Time after last sample in clock tics"
  Clock at Sample Time/1 -> Sum1/2  "Time in delt multiples"
  Clock at tics/1 -> Sum1/1  "Time in clockt multiples"
  ton/1 -> Sum/1  "ton"
  Constant/1 -> Relational Operator/2

== system Final_Project_EEM_EKF_SIM/Reaction Jet Control/Reaction Jet Control/v Control Law/Subsystem ==
  note: Firefct1
      | This function establishes when the jets are to be fired in a negative sense
      | Firefct1 = e + edot ^2/(2*N*alph) - DB
  e and edot : Inport
  NofJets : Inport  Port=2
  1/(2*alph) : Gain  Gain=1/(2*alph)  SaturateOnIntegerOverflow=on  OutDataTypeStr=Inherit: Same as input  ParamDataTypeStr=Inherit: Same as input
  Constant2 : Constant  Value=DB
  Select e : Selector  InputPortWidth=2  IndexOptions=Index vector (dialog)  Indices=[1]  OutputSizes=1
  Select edot : Selector  InputPortWidth=2  IndexOptions=Index vector (dialog)  Indices=[2]  OutputSizes=1
  Sum1 : Sum  Inputs=-++  InputSameDT=on  SaturateOnIntegerOverflow=on  OutDataTypeStr=Inherit: Same as first input
  edot^2 : Product  Inputs=/**  InputSameDT=on  RndMeth=Zero  SaturateOnIntegerOverflow=on  OutDataTypeStr=Inherit: Same as first input
  Firefct1 : Outport  VectorParamsAs1DForOutWhenUnconnected=off
  wires:
  Sum1/1 -> Firefct1/1
  Select e/1 -> Sum1/2  "e"
  Constant2/1 -> Sum1/1
  1/(2*alph)/1 -> Sum1/3
  e and edot/1 -> Select edot/1, Select e/1
  NofJets/1 -> edot^2/1
  Select edot/1 -> edot^2/3, edot^2/2  "edot"
  edot^2/1 -> 1/(2*alph)/1  "edot^2"

== system Final_Project_EEM_EKF_SIM/Reaction Jet Control/Reaction Jet Control/v Control Law/Subsystem1 ==
  note: Coastfct1
      | This function establishes when the jets are to be turned off (coasting)
      | Coastfct1 = e - edot ^2/(2*N*alphs) - DB
  e and edot : Inport
  NofJets : Inport  Port=2
  1/(2*alph) : Gain  Gain=1/(2*alphs)  SaturateOnIntegerOverflow=on  OutDataTypeStr=Inherit: Same as input  ParamDataTypeStr=Inherit: Same as input
  Constant2 : Constant  Value=DB
  Select e : Selector  InputPortWidth=2  IndexOptions=Index vector (dialog)  Indices=[1]  OutputSizes=1
  Select edot : Selector  InputPortWidth=2  IndexOptions=Index vector (dialog)  Indices=[2]  OutputSizes=1
  Sum1 : Sum  Inputs=-+-  InputSameDT=on  SaturateOnIntegerOverflow=on  OutDataTypeStr=Inherit: Same as first input
  edot^2 : Product  Inputs=/**  InputSameDT=on  RndMeth=Zero  SaturateOnIntegerOverflow=on  OutDataTypeStr=Inherit: Same as first input
  Coastfct1 : Outport  VectorParamsAs1DForOutWhenUnconnected=off
  wires:
  edot^2/1 -> 1/(2*alph)/1  "edot^2"
  Select edot/1 -> edot^2/2, edot^2/3  "edot"
  NofJets/1 -> edot^2/1
  e and edot/1 -> Select e/1, Select edot/1
  1/(2*alph)/1 -> Sum1/3
  Constant2/1 -> Sum1/1
  Select e/1 -> Sum1/2  "e"
  Sum1/1 -> Coastfct1/1

== system Final_Project_EEM_EKF_SIM/Reaction Jet Control/Reaction Jet Control/v Control Law/Subsystem2 ==
  note: Firefct2
      | This function establishes when the jets are to be fired in a positive sense
      | Firefct2 = e - edot ^2/(2*N*alph) + DB
  e and edot : Inport
  NofJets : Inport  Port=2
  1/(2*alph) : Gain  Gain=1/(2*alph)  SaturateOnIntegerOverflow=on  OutDataTypeStr=Inherit: Same as input  ParamDataTypeStr=Inherit: Same as input
  Constant2 : Constant  Value=DB
  Select e : Selector  InputPortWidth=2  IndexOptions=Index vector (dialog)  Indices=[1]  OutputSizes=1
  Select edot : Selector  InputPortWidth=2  IndexOptions=Index vector (dialog)  Indices=[2]  OutputSizes=1
  Sum1 : Sum  Inputs=++-  InputSameDT=on  SaturateOnIntegerOverflow=on  OutDataTypeStr=Inherit: Same as first input
  edot^2 : Product  Inputs=/**  InputSameDT=on  RndMeth=Zero  SaturateOnIntegerOverflow=on  OutDataTypeStr=Inherit: Same as first input
  Firefct2 : Outport  VectorParamsAs1DForOutWhenUnconnected=off
  wires:
  Sum1/1 -> Firefct2/1
  Select e/1 -> Sum1/2  "e"
  Constant2/1 -> Sum1/1
  1/(2*alph)/1 -> Sum1/3
  e and edot/1 -> Select edot/1, Select e/1
  NofJets/1 -> edot^2/1
  Select edot/1 -> edot^2/3, edot^2/2  "edot"
  edot^2/1 -> 1/(2*alph)/1  "edot^2"

== system Final_Project_EEM_EKF_SIM/Reaction Jet Control/Reaction Jet Control/v Control Law/Subsystem3 ==
  note: Coastfct2
      | This function establishes when the jets are to be turned off (coasting)
      | Coastfct1 = e + edot ^2/(2*N*alphs) + DB
  e and edot : Inport
  NofJets : Inport  Port=2
  1/(2*alph) : Gain  Gain=1/(2*alphs)  SaturateOnIntegerOverflow=on  OutDataTypeStr=Inherit: Same as input  ParamDataTypeStr=Inherit: Same as input
  Constant2 : Constant  Value=DB
  Select e : Selector  InputPortWidth=2  IndexOptions=Index vector (dialog)  Indices=[1]  OutputSizes=1
  Select edot : Selector  InputPortWidth=2  IndexOptions=Index vector (dialog)  Indices=[2]  OutputSizes=1
  Sum1 : Sum  Inputs=+++  InputSameDT=on  SaturateOnIntegerOverflow=on  OutDataTypeStr=Inherit: Same as first input
  edot^2 : Product  Inputs=/**  InputSameDT=on  RndMeth=Zero  SaturateOnIntegerOverflow=on  OutDataTypeStr=Inherit: Same as first input
  Coastfct2 : Outport  VectorParamsAs1DForOutWhenUnconnected=off
  wires:
  Sum1/1 -> Coastfct2/1
  Select e/1 -> Sum1/2  "e"
  Constant2/1 -> Sum1/1
  1/(2*alph)/1 -> Sum1/3
  e and edot/1 -> Select edot/1, Select e/1
  NofJets/1 -> edot^2/1
  Select edot/1 -> edot^2/3, edot^2/2  "edot"
  edot^2/1 -> 1/(2*alph)/1  "edot^2"

== stateflow chart Final_Project_EEM_EKF_SIM/Reaction Jet Control/Reaction Jet Control/u Control Law/Chart ==
  settings: updateMethod=DISCRETE  sampleTime=delt
  state Wait_for_stable_rate
  state Start
  state Fire_region_1
    en: jets=-Nofjets;
    ton=tjcalc+tjcalc1;
  state Coast_region_2
    en: jets=0;
    ton=0;
    enable=0;
  state Skip_a_Sample_2
    en:count--;
  state Skip_a_Sample_1
    en:count--;
  state Coast_region_1
    en: jets=0;
    ton=0;
    enable=0;
  state Fire_region_2
    en: jets=Nofjets;
    ton=tjcalc-tjcalc1;
  Wait_for_stable_rate -> Start [order 1] : [count==0]
  (default) -> Wait_for_stable_rate : /count=2;
  Wait_for_stable_rate -> Wait_for_stable_rate [order 2] : /count--;
  Start -> Fire_region_2 [order 1] : [ (e[1]<0 & Firefct2<0) | (e[1]>0 & Coastfct2>0) ]
  Start -> Coast_region_1 [order 4] : [ (e[1]<0 & Coastfct1<=0 & Firefct2>0) ]
  Start -> Coast_region_2 [order 2] : [ (e[1]>0 & Coastfct2>=0 & Firefct1<0) ]
  Start -> Fire_region_1 [order 3] : [ (e[1]>0 & Firefct1>0) | (e[1]<0 & Coastfct1<0) ]
  Coast_region_2 -> Fire_region_1 : [e[1]>0 & Firefct1>0]
  Skip_a_Sample_2 -> Coast_region_2 [order 1] : [count==0]
  Fire_region_1 -> (junction 32) [order 2] : [ton<2*delt]{enable=1;}
  Fire_region_1 -> Coast_region_1 [order 1] : [e[1]<0 & Coastfct1<=0]
  Fire_region_1 -> Fire_region_1 [order 3]
  (junction 33) -> Coast_region_2 [order 2] : {enable=0;}
  Fire_region_2 -> Coast_region_2 [order 2] : [e[1]>0 & Coastfct2>0]
  (junction 32) -> Coast_region_1 [order 2] : {enable=0;}
  (junction 32) -> Skip_a_Sample_1 [order 1] : [ton>tmin]{count=2;}
  Skip_a_Sample_2 -> Skip_a_Sample_2 [order 2] : /ton=ton-delt;
  (junction 33) -> Skip_a_Sample_2 [order 1] : [ton>tmin]{count=2;}
  Skip_a_Sample_1 -> Skip_a_Sample_1 [order 2] : /ton=ton-delt;
  Skip_a_Sample_1 -> Coast_region_1 [order 1] : [count==0]
  Fire_region_2 -> (junction 33) [order 1] : [ton<2*delt]{enable=1;}
  Coast_region_1 -> Fire_region_2 : [e[1]<0 & Firefct2<0]
  Fire_region_2 -> Fire_region_2 [order 3]
  data: jets output double; Nofjets input double; e input double size=2; enable output boolean; ton output double; Firefct1 input double; Coastfct1 input double; Firefct2 input double; Coastfct2 input double; tjcalc1 input double; tjcalc input double; tmin parameter double; delt parameter double; count local double

== stateflow chart Final_Project_EEM_EKF_SIM/Reaction Jet Control/Reaction Jet Control/Yaw Control Law/Chart ==
  settings: updateMethod=DISCRETE  sampleTime=delt
  state Wait_for_stable_rate
  state Start
  state Fire_region_1
    en: jets=-Nofjets;
    ton=tjcalc+tjcalc1;
  state Coast_region_2
    en: jets=0;
    ton=0;
    enable=0;
  state Skip_a_Sample_2
    en:count--;
  state Skip_a_Sample_1
    en:count--;
  state Coast_region_1
    en: jets=0;
    ton=0;
    enable=0;
  state Fire_region_2
    en: jets=Nofjets;
    ton=tjcalc-tjcalc1;
  Wait_for_stable_rate -> Start [order 1] : [count==0]
  (default) -> Wait_for_stable_rate : /count=2;
  Wait_for_stable_rate -> Wait_for_stable_rate [order 2] : /count--;
  Start -> Fire_region_2 [order 1] : [ (e[1]<0 & Firefct2<0) | (e[1]>0 & Coastfct2>0) ]
  Start -> Coast_region_1 [order 4] : [ (e[1]<0 & Coastfct1<=0 & Firefct2>0) ]
  Start -> Coast_region_2 [order 2] : [ (e[1]>0 & Coastfct2>=0 & Firefct1<0) ]
  Start -> Fire_region_1 [order 3] : [ (e[1]>0 & Firefct1>0) | (e[1]<0 & Coastfct1<0) ]
  Coast_region_2 -> Fire_region_1 : [e[1]>0 & Firefct1>0]
  Skip_a_Sample_2 -> Coast_region_2 [order 1] : [count==0]
  Fire_region_1 -> (junction 32) [order 2] : [ton<2*delt]{enable=1;}
  Fire_region_1 -> Coast_region_1 [order 1] : [e[1]<0 & Coastfct1<=0]
  Fire_region_1 -> Fire_region_1 [order 3]
  (junction 33) -> Coast_region_2 [order 2] : {enable=0;}
  Fire_region_2 -> Coast_region_2 [order 2] : [e[1]>0 & Coastfct2>0]
  (junction 32) -> Coast_region_1 [order 2] : {enable=0;}
  (junction 32) -> Skip_a_Sample_1 [order 1] : [ton>tmin]{count=2;}
  Skip_a_Sample_2 -> Skip_a_Sample_2 [order 2] : /ton=ton-delt;
  (junction 33) -> Skip_a_Sample_2 [order 1] : [ton>tmin]{count=2;}
  Skip_a_Sample_1 -> Skip_a_Sample_1 [order 2] : /ton=ton-delt;
  Skip_a_Sample_1 -> Coast_region_1 [order 1] : [count==0]
  Fire_region_2 -> (junction 33) [order 1] : [ton<2*delt]{enable=1;}
  Coast_region_1 -> Fire_region_2 : [e[1]<0 & Firefct2<0]
  Fire_region_2 -> Fire_region_2 [order 3]
  data: jets output double; Nofjets input double; e input double size=2; enable output boolean; ton output double; Firefct1 input double; Coastfct1 input double; Firefct2 input double; Coastfct2 input double; tjcalc1 input double; tjcalc input double; tmin parameter double; delt parameter double; count local double

== stateflow chart Final_Project_EEM_EKF_SIM/Reaction Jet Control/Reaction Jet Control/v Control Law/Chart ==
  settings: updateMethod=DISCRETE  sampleTime=delt
  state Wait_for_stable_rate
  state Start
  state Fire_region_1
    en: jets=-Nofjets;
    ton=tjcalc+tjcalc1;
  state Coast_region_2
    en: jets=0;
    ton=0;
    enable=0;
  state Skip_a_Sample_2
    en:count--;
  state Skip_a_Sample_1
    en:count--;
  state Coast_region_1
    en: jets=0;
    ton=0;
    enable=0;
  state Fire_region_2
    en: jets=Nofjets;
    ton=tjcalc-tjcalc1;
  Wait_for_stable_rate -> Start [order 1] : [count==0]
  (default) -> Wait_for_stable_rate : /count=2;
  Wait_for_stable_rate -> Wait_for_stable_rate [order 2] : /count--;
  Start -> Fire_region_2 [order 1] : [ (e[1]<0 & Firefct2<0) | (e[1]>0 & Coastfct2>0) ]
  Start -> Coast_region_1 [order 4] : [ (e[1]<0 & Coastfct1<=0 & Firefct2>0) ]
  Start -> Coast_region_2 [order 2] : [ (e[1]>0 & Coastfct2>=0 & Firefct1<0) ]
  Start -> Fire_region_1 [order 3] : [ (e[1]>0 & Firefct1>0) | (e[1]<0 & Coastfct1<0) ]
  Coast_region_2 -> Fire_region_1 : [e[1]>0 & Firefct1>0]
  Skip_a_Sample_2 -> Coast_region_2 [order 1] : [count==0]
  Fire_region_1 -> (junction 32) [order 2] : [ton<2*delt]{enable=1;}
  Fire_region_1 -> Coast_region_1 [order 1] : [e[1]<0 & Coastfct1<=0]
  Fire_region_1 -> Fire_region_1 [order 3]
  (junction 33) -> Coast_region_2 [order 2] : {enable=0;}
  Fire_region_2 -> Coast_region_2 [order 2] : [e[1]>0 & Coastfct2>0]
  (junction 32) -> Coast_region_1 [order 2] : {enable=0;}
  (junction 32) -> Skip_a_Sample_1 [order 1] : [ton>tmin]{count=2;}
  Skip_a_Sample_2 -> Skip_a_Sample_2 [order 2] : /ton=ton-delt;
  (junction 33) -> Skip_a_Sample_2 [order 1] : [ton>tmin]{count=2;}
  Skip_a_Sample_1 -> Skip_a_Sample_1 [order 2] : /ton=ton-delt;
  Skip_a_Sample_1 -> Coast_region_1 [order 1] : [count==0]
  Fire_region_2 -> (junction 33) [order 1] : [ton<2*delt]{enable=1;}
  Coast_region_1 -> Fire_region_2 : [e[1]<0 & Firefct2<0]
  Fire_region_2 -> Fire_region_2 [order 3]
  data: jets output double; Nofjets input double; e input double size=2; enable output boolean; ton output double; Firefct1 input double; Coastfct1 input double; Firefct2 input double; Coastfct2 input double; tjcalc1 input double; tjcalc input double; tmin parameter double; delt parameter double; count local double
